simulink model "Questao3"  (R2017b)
settings: Solver=VariableStepAuto  StartTime=0.0  StopTime=100  RelTol=1e-3
values from neighbouring files (symbols this model uses):
  Cz = tf(Cz)    [main.m]
  Fz = tf(Fz)    [main.m]
  Gz = c2d(Gs,T)    [main.m]
  Hz = c2d(Hs,T)    [main.m]
  Pz = c2d(Ps,T)    [main.m]
  T = 0.1    [main.m]
libraries: simulink x2
settings Model: Creator=mathe_tykk233  LastModifiedBy=mathe_tykk233

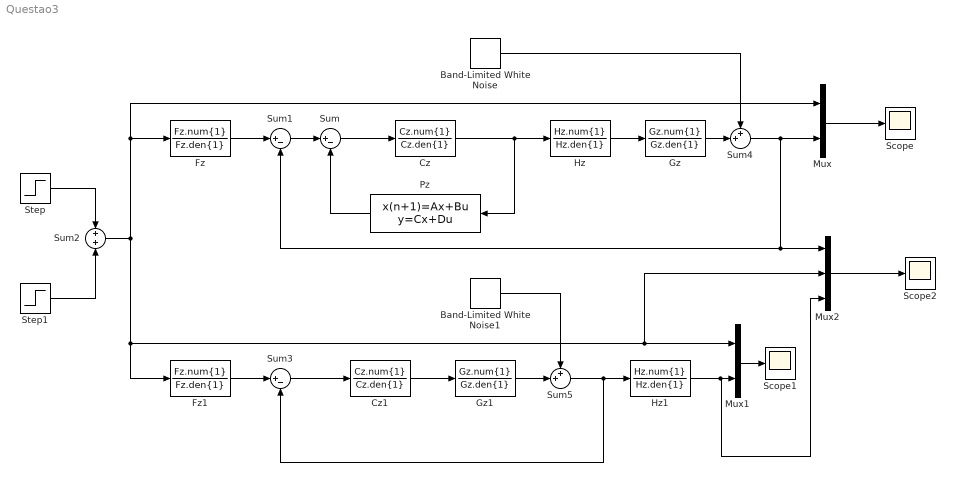
== system Questao3 ==
  Band-Limited White Noise : simulink/Sources/Band-Limited White Noise  Cov=1e-7  Ts=1e-3  seed=[23341]
  Band-Limited White Noise1 : simulink/Sources/Band-Limited White Noise  Cov=1e-7  Ts=1e-3  seed=[23341]
  Cz : DiscreteTransferFcn  Numerator=Cz.num{1}  Denominator=Cz.den{1}  SampleTime=T
  Cz1 : DiscreteTransferFcn  Numerator=Cz.num{1}  Denominator=Cz.den{1}  SampleTime=T
  Fz : DiscreteTransferFcn  Numerator=Fz.num{1}  Denominator=Fz.den{1}  SampleTime=T
  Fz1 : DiscreteTransferFcn  Numerator=Fz.num{1}  Denominator=Fz.den{1}  SampleTime=T
  Gz : DiscreteTransferFcn  Numerator=Gz.num{1}  Denominator=Gz.den{1}  SampleTime=T
  Gz1 : DiscreteTransferFcn  Numerator=Gz.num{1}  Denominator=Gz.den{1}  SampleTime=T
  Hz : DiscreteTransferFcn  Numerator=Hz.num{1}  Denominator=Hz.den{1}  SampleTime=T
  Hz1 : DiscreteTransferFcn  Numerator=Hz.num{1}  Denominator=Hz.den{1}  SampleTime=T
  Mux : Mux  Inputs=2
  Mux1 : Mux  Inputs=2
  Mux2 : Mux  Inputs=3
  Pz : DiscreteStateSpace  A=Pz.A  B=Pz.B  C=Pz.C  D=Pz.D  SampleTime=T
  Scope : Scope
  Scope1 : Scope
  Scope2 : Scope
  Step : Step  Time=60  After=-0.5  SampleTime=0
  Step1 : Step  SampleTime=0
  Sum : Sum  Inputs=|+-
  Sum1 : Sum  Inputs=|+-
  Sum2 : Sum  Inputs=+|+
  Sum3 : Sum  Inputs=|+-
  Sum4 : Sum  Inputs=++|
  Sum5 : Sum  Inputs=++|
  wires:
  Cz/1 -> Pz/1, Hz/1
  Sum/1 -> Cz/1
  Pz/1 -> Sum/2
  Sum1/1 -> Sum/1
  Fz/1 -> Sum1/1
  Sum2/1 -> Fz1/1, Mux2/2, Mux1/1, Mux/1, Fz/1
  Mux/1 -> Scope/1
  Fz1/1 -> Sum3/1
  Mux1/1 -> Scope1/1
  Hz1/1 -> Mux2/3, Mux1/2
  Sum3/1 -> Cz1/1
  Cz1/1 -> Gz1/1
  Mux2/1 -> Scope2/1
  Step/1 -> Sum2/1
  Step1/1 -> Sum2/2
  Band-Limited White Noise/1 -> Sum4/1
  Hz/1 -> Gz/1
  Gz/1 -> Sum4/2
  Sum4/1 -> Mux2/1, Sum1/2, Mux/2
  Gz1/1 -> Sum5/2
  Sum5/1 -> Sum3/2, Hz1/1
  Band-Limited White Noise1/1 -> Sum5/1
